simulink model "AUV_6DoF"  (R2020b)
settings: Solver=VariableStepAuto  StartTime=0.0  StopTime=60  RelTol=1e-3
libraries: pid_lib x4, simulink x1
settings Model: Creator=shanerutherford  LastModifiedBy=shanerutherford

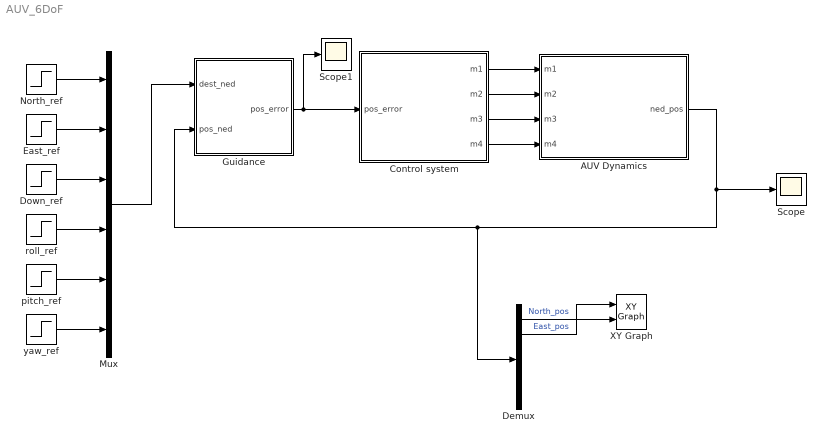
== system AUV_6DoF ==
  AUV Dynamics : Subsystem
  Control system : Subsystem
  Demux : Demux  Outputs=6
  Down_ref : Step  Time=0  After=0  SampleTime=0
  East_ref : Step  Time=0  After=-1  SampleTime=0
  Guidance : MATLAB Function  TreatAsAtomicUnit=on
  Mux : Mux  Inputs=6
  North_ref : Step  Time=0  After=-1  SampleTime=0
  Scope : Scope
  Scope1 : Scope
  XY Graph : simulink/Sinks/XY Graph  xmin=-10  xmax=10  ymin=-10  ymax=10  st=-1
  pitch_ref : Step  Time=0  After=0  SampleTime=0
  roll_ref : Step  Time=0  After=0  SampleTime=0
  yaw_ref : Step  Time=0  After=0  SampleTime=0
  wires:
  Control system/1(m1) -> AUV Dynamics/1(m1)
  Control system/2(m2) -> AUV Dynamics/2(m2)
  Control system/3(m3) -> AUV Dynamics/3(m3)
  Control system/4(m4) -> AUV Dynamics/4(m4)
  Guidance/1(pos_error) -> Scope1/1, Control system/1(pos_error)
  Mux/1 -> Guidance/1(dest_ned)
  North_ref/1 -> Mux/1
  Down_ref/1 -> Mux/3
  roll_ref/1 -> Mux/4
  yaw_ref/1 -> Mux/6
  East_ref/1 -> Mux/2
  pitch_ref/1 -> Mux/5
  AUV Dynamics/1(ned_pos) -> Scope/1, Demux/1, Guidance/2(pos_ned)
  Demux/1 -> XY Graph/2  "North_pos"
  Demux/2 -> XY Graph/1  "East_pos"

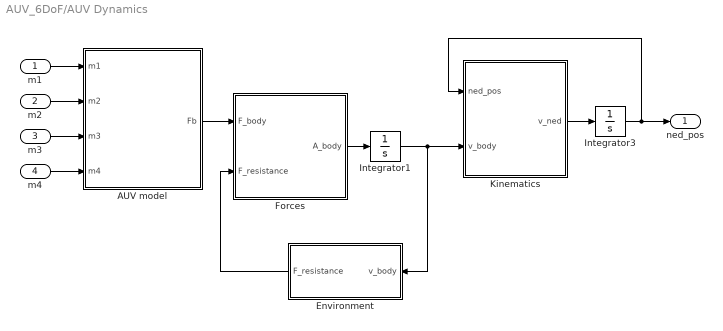
== system AUV_6DoF/AUV Dynamics ==
  m1 : Inport
  m2 : Inport  Port=2
  m3 : Inport  Port=3
  m4 : Inport  Port=4
  AUV model : MATLAB Function  TreatAsAtomicUnit=on
  Environment : MATLAB Function  TreatAsAtomicUnit=on
  Forces : MATLAB Function  TreatAsAtomicUnit=on
  Integrator1 : Integrator
  Integrator3 : Integrator
  Kinematics : MATLAB Function  TreatAsAtomicUnit=on
  ned_pos : Outport  PortDimensions=6
  wires:
  m1/1 -> AUV model/1(m1)
  m2/1 -> AUV model/2(m2)
  m3/1 -> AUV model/3(m3)
  m4/1 -> AUV model/4(m4)
  Integrator3/1 -> ned_pos/1, Kinematics/1(ned_pos)
  Kinematics/1(v_ned) -> Integrator3/1
  AUV model/1(Fb) -> Forces/1(F_body)
  Environment/1(F_resistance) -> Forces/2(F_resistance)
  Forces/1(A_body) -> Integrator1/1
  Integrator1/1 -> Kinematics/2(v_body), Environment/1(v_body)

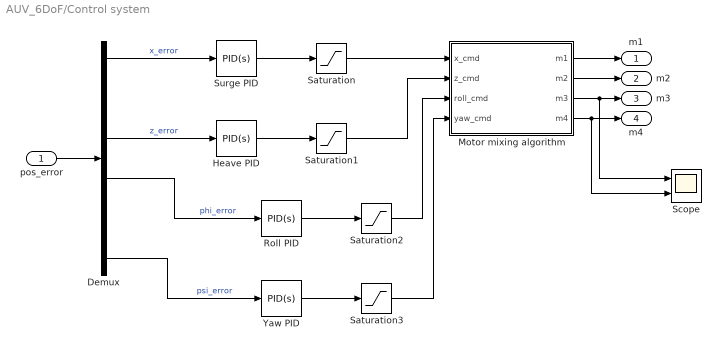
== system AUV_6DoF/Control system ==
  pos_error : Inport
  Demux : Demux  Outputs=6
  Heave PID : pid_lib/PID Controller  Controller=PID  Form=Parallel  TimeDomain=Continuous-time  UseExternalTs=off  SampleTime=-1  IntegratorMethod=Forward Euler  FilterMethod=Forward Euler  ControllerParametersSource=internal  P=1  I=0  D=5  UseFilter=on  N=100  TunerSelectOption=Transfer Function Based (PID Tuner App)  InitialConditionSource=internal  InitialConditionForIntegrator=0  InitialConditionForFilter=0  DifferentiatorICPrevScaledInput=0  ExternalReset=none  TrackingMode=off  Kt=1  LimitOutput=off  SatLimitsSource=internal  UpperSaturationLimit=inf  LowerSaturationLimit=-inf  LinearizeAsGain=on  AntiWindupMode=none  Kb=1  POutMin=[]  POutMax=[]  IOutMin=[]  IOutMax=[]  DOutMin=[]  DOutMax=[]  NOutMin=[]  NOutMax=[]  SumOutMin=[]  SumOutMax=[]  SaturationOutMin=[]  SaturationOutMax=[]  PParamMin=[]  PParamMax=[]  IParamMin=[]  IParamMax=[]  DParamMin=[]  DParamMax=[]  NParamMin=[]  NParamMax=[]  KbParamMin=[]  KbParamMax=[]  KtParamMin=[]  KtParamMax=[]  KbOutMin=[]  KbOutMax=[]  KtOutMin=[]  KtOutMax=[]  IntegratorOutMin=[]  IntegratorOutMax=[]  FilterOutMin=[]  FilterOutMax=[]  SumI1OutMin=[]  SumI1OutMax=[]  SumI2OutMin=[]  SumI2OutMax=[]  SumI3OutMin=[]  SumI3OutMax=[]  SumI4OutMin=[]  SumI4OutMax=[]  SumDOutMin=[]  SumDOutMax=[]  DifferentiatorOutMin=[]  DifferentiatorOutMax=[]  FilterDiffOutCoefMin=[]  FilterDiffOutCoefMax=[]  ReciprocalOutMin=[]  ReciprocalOutMax=[]  SumDenOutMin=[]  SumDenOutMax=[]  SumNumOutMin=[]  SumNumOutMax=[]  DivideOutMin=[]  DivideOutMax=[]  UdiffTsProdOutMin=[]  UdiffTsProdOutMax=[]  NTsProdOutMin=[]  NTsProdOutMax=[]  UintegralTsProdOutMin=[]  UintegralTsProdOutMax=[]  UngainTsProdOutMin=[]  UngainTsProdOutMax=[]  IntegratorContinuousStateAttributes=''  IntegratorStateMustResolveToSignalObject=off  IntegratorRTWStateStorageClass=Auto  FilterContinuousStateAttributes=''  FilterStateMustResolveToSignalObject=off  FilterRTWStateStorageClass=Auto  ParallelPVariant=InternalParameters  IdealPVariant=Disabled  IVariant=InternalParameters  DVariant=InternalParameters  IntegratorVariant=Continuous  SatVariant=Disabled  AWVariant=Passthrough  PCopyVariant=Disabled  TRVariant=Disabled  FdbkBlocksVariant=Forward  IdealPFdbkVariant=Disabled  SatFdbkVariant=Disabled  DerivativeFilterVariant=ContFilter  NVariant=InternalParameters  NCopyVariant=Disabled  FilterICVariant=InternalICsFilter  IntegratorICVariant=InternalICs  ExternalResetVariant=Disabled  TRSumVariant=Passthrough  SumFdbkVariant=Disabled  SumVariant=Sum_PID  TsampFilterVariant=InternalTs  TsampNgainVariant=Passthrough  TsampIntegralVariant=Passthrough  ExternalSaturationOutDataTypeStr=Inherit: Same as second input
  Motor mixing algorithm : MATLAB Function  TreatAsAtomicUnit=on
  Roll PID : pid_lib/PID Controller  Controller=PID  Form=Parallel  TimeDomain=Continuous-time  UseExternalTs=off  SampleTime=-1  IntegratorMethod=Forward Euler  FilterMethod=Forward Euler  ControllerParametersSource=internal  P=1  I=0  D=5  UseFilter=on  N=100  TunerSelectOption=Transfer Function Based (PID Tuner App)  InitialConditionSource=internal  InitialConditionForIntegrator=0  InitialConditionForFilter=0  DifferentiatorICPrevScaledInput=0  ExternalReset=none  TrackingMode=off  Kt=1  LimitOutput=off  SatLimitsSource=internal  UpperSaturationLimit=inf  LowerSaturationLimit=-inf  LinearizeAsGain=on  AntiWindupMode=none  Kb=1  POutMin=[]  POutMax=[]  IOutMin=[]  IOutMax=[]  DOutMin=[]  DOutMax=[]  NOutMin=[]  NOutMax=[]  SumOutMin=[]  SumOutMax=[]  SaturationOutMin=[]  SaturationOutMax=[]  PParamMin=[]  PParamMax=[]  IParamMin=[]  IParamMax=[]  DParamMin=[]  DParamMax=[]  NParamMin=[]  NParamMax=[]  KbParamMin=[]  KbParamMax=[]  KtParamMin=[]  KtParamMax=[]  KbOutMin=[]  KbOutMax=[]  KtOutMin=[]  KtOutMax=[]  IntegratorOutMin=[]  IntegratorOutMax=[]  FilterOutMin=[]  FilterOutMax=[]  SumI1OutMin=[]  SumI1OutMax=[]  SumI2OutMin=[]  SumI2OutMax=[]  SumI3OutMin=[]  SumI3OutMax=[]  SumI4OutMin=[]  SumI4OutMax=[]  SumDOutMin=[]  SumDOutMax=[]  DifferentiatorOutMin=[]  DifferentiatorOutMax=[]  FilterDiffOutCoefMin=[]  FilterDiffOutCoefMax=[]  ReciprocalOutMin=[]  ReciprocalOutMax=[]  SumDenOutMin=[]  SumDenOutMax=[]  SumNumOutMin=[]  SumNumOutMax=[]  DivideOutMin=[]  DivideOutMax=[]  UdiffTsProdOutMin=[]  UdiffTsProdOutMax=[]  NTsProdOutMin=[]  NTsProdOutMax=[]  UintegralTsProdOutMin=[]  UintegralTsProdOutMax=[]  UngainTsProdOutMin=[]  UngainTsProdOutMax=[]  IntegratorContinuousStateAttributes=''  IntegratorStateMustResolveToSignalObject=off  IntegratorRTWStateStorageClass=Auto  FilterContinuousStateAttributes=''  FilterStateMustResolveToSignalObject=off  FilterRTWStateStorageClass=Auto  ParallelPVariant=InternalParameters  IdealPVariant=Disabled  IVariant=InternalParameters  DVariant=InternalParameters  IntegratorVariant=Continuous  SatVariant=Disabled  AWVariant=Passthrough  PCopyVariant=Disabled  TRVariant=Disabled  FdbkBlocksVariant=Forward  IdealPFdbkVariant=Disabled  SatFdbkVariant=Disabled  DerivativeFilterVariant=ContFilter  NVariant=InternalParameters  NCopyVariant=Disabled  FilterICVariant=InternalICsFilter  IntegratorICVariant=InternalICs  ExternalResetVariant=Disabled  TRSumVariant=Passthrough  SumFdbkVariant=Disabled  SumVariant=Sum_PID  TsampFilterVariant=InternalTs  TsampNgainVariant=Passthrough  TsampIntegralVariant=Passthrough  ExternalSaturationOutDataTypeStr=Inherit: Same as second input
  Saturation{,1..3} (4 alike) : Saturate  UpperLimit=0.3  LowerLimit=-0.3
  Scope : Scope  NumInputPorts=2
  Surge PID : pid_lib/PID Controller  Controller=PID  Form=Parallel  TimeDomain=Continuous-time  UseExternalTs=off  SampleTime=-1  IntegratorMethod=Forward Euler  FilterMethod=Forward Euler  ControllerParametersSource=internal  P=1  I=0  D=5  UseFilter=on  N=100  TunerSelectOption=Transfer Function Based (PID Tuner App)  InitialConditionSource=internal  InitialConditionForIntegrator=0  InitialConditionForFilter=0  DifferentiatorICPrevScaledInput=0  ExternalReset=none  TrackingMode=off  Kt=1  LimitOutput=off  SatLimitsSource=internal  UpperSaturationLimit=inf  LowerSaturationLimit=-inf  LinearizeAsGain=on  AntiWindupMode=none  Kb=1  POutMin=[]  POutMax=[]  IOutMin=[]  IOutMax=[]  DOutMin=[]  DOutMax=[]  NOutMin=[]  NOutMax=[]  SumOutMin=[]  SumOutMax=[]  SaturationOutMin=[]  SaturationOutMax=[]  PParamMin=[]  PParamMax=[]  IParamMin=[]  IParamMax=[]  DParamMin=[]  DParamMax=[]  NParamMin=[]  NParamMax=[]  KbParamMin=[]  KbParamMax=[]  KtParamMin=[]  KtParamMax=[]  KbOutMin=[]  KbOutMax=[]  KtOutMin=[]  KtOutMax=[]  IntegratorOutMin=[]  IntegratorOutMax=[]  FilterOutMin=[]  FilterOutMax=[]  SumI1OutMin=[]  SumI1OutMax=[]  SumI2OutMin=[]  SumI2OutMax=[]  SumI3OutMin=[]  SumI3OutMax=[]  SumI4OutMin=[]  SumI4OutMax=[]  SumDOutMin=[]  SumDOutMax=[]  DifferentiatorOutMin=[]  DifferentiatorOutMax=[]  FilterDiffOutCoefMin=[]  FilterDiffOutCoefMax=[]  ReciprocalOutMin=[]  ReciprocalOutMax=[]  SumDenOutMin=[]  SumDenOutMax=[]  SumNumOutMin=[]  SumNumOutMax=[]  DivideOutMin=[]  DivideOutMax=[]  UdiffTsProdOutMin=[]  UdiffTsProdOutMax=[]  NTsProdOutMin=[]  NTsProdOutMax=[]  UintegralTsProdOutMin=[]  UintegralTsProdOutMax=[]  UngainTsProdOutMin=[]  UngainTsProdOutMax=[]  IntegratorContinuousStateAttributes=''  IntegratorStateMustResolveToSignalObject=off  IntegratorRTWStateStorageClass=Auto  FilterContinuousStateAttributes=''  FilterStateMustResolveToSignalObject=off  FilterRTWStateStorageClass=Auto  ParallelPVariant=InternalParameters  IdealPVariant=Disabled  IVariant=InternalParameters  DVariant=InternalParameters  IntegratorVariant=Continuous  SatVariant=Disabled  AWVariant=Passthrough  PCopyVariant=Disabled  TRVariant=Disabled  FdbkBlocksVariant=Forward  IdealPFdbkVariant=Disabled  SatFdbkVariant=Disabled  DerivativeFilterVariant=ContFilter  NVariant=InternalParameters  NCopyVariant=Disabled  FilterICVariant=InternalICsFilter  IntegratorICVariant=InternalICs  ExternalResetVariant=Disabled  TRSumVariant=Passthrough  SumFdbkVariant=Disabled  SumVariant=Sum_PID  TsampFilterVariant=InternalTs  TsampNgainVariant=Passthrough  TsampIntegralVariant=Passthrough  ExternalSaturationOutDataTypeStr=Inherit: Same as second input
  Yaw PID : pid_lib/PID Controller  Controller=PID  Form=Parallel  TimeDomain=Continuous-time  UseExternalTs=off  SampleTime=-1  IntegratorMethod=Forward Euler  FilterMethod=Forward Euler  ControllerParametersSource=internal  P=1  I=0  D=5  UseFilter=on  N=100  TunerSelectOption=Transfer Function Based (PID Tuner App)  InitialConditionSource=internal  InitialConditionForIntegrator=0  InitialConditionForFilter=0  DifferentiatorICPrevScaledInput=0  ExternalReset=none  TrackingMode=off  Kt=1  LimitOutput=off  SatLimitsSource=internal  UpperSaturationLimit=inf  LowerSaturationLimit=-inf  LinearizeAsGain=on  AntiWindupMode=none  Kb=1  POutMin=[]  POutMax=[]  IOutMin=[]  IOutMax=[]  DOutMin=[]  DOutMax=[]  NOutMin=[]  NOutMax=[]  SumOutMin=[]  SumOutMax=[]  SaturationOutMin=[]  SaturationOutMax=[]  PParamMin=[]  PParamMax=[]  IParamMin=[]  IParamMax=[]  DParamMin=[]  DParamMax=[]  NParamMin=[]  NParamMax=[]  KbParamMin=[]  KbParamMax=[]  KtParamMin=[]  KtParamMax=[]  KbOutMin=[]  KbOutMax=[]  KtOutMin=[]  KtOutMax=[]  IntegratorOutMin=[]  IntegratorOutMax=[]  FilterOutMin=[]  FilterOutMax=[]  SumI1OutMin=[]  SumI1OutMax=[]  SumI2OutMin=[]  SumI2OutMax=[]  SumI3OutMin=[]  SumI3OutMax=[]  SumI4OutMin=[]  SumI4OutMax=[]  SumDOutMin=[]  SumDOutMax=[]  DifferentiatorOutMin=[]  DifferentiatorOutMax=[]  FilterDiffOutCoefMin=[]  FilterDiffOutCoefMax=[]  ReciprocalOutMin=[]  ReciprocalOutMax=[]  SumDenOutMin=[]  SumDenOutMax=[]  SumNumOutMin=[]  SumNumOutMax=[]  DivideOutMin=[]  DivideOutMax=[]  UdiffTsProdOutMin=[]  UdiffTsProdOutMax=[]  NTsProdOutMin=[]  NTsProdOutMax=[]  UintegralTsProdOutMin=[]  UintegralTsProdOutMax=[]  UngainTsProdOutMin=[]  UngainTsProdOutMax=[]  IntegratorContinuousStateAttributes=''  IntegratorStateMustResolveToSignalObject=off  IntegratorRTWStateStorageClass=Auto  FilterContinuousStateAttributes=''  FilterStateMustResolveToSignalObject=off  FilterRTWStateStorageClass=Auto  ParallelPVariant=InternalParameters  IdealPVariant=Disabled  IVariant=InternalParameters  DVariant=InternalParameters  IntegratorVariant=Continuous  SatVariant=Disabled  AWVariant=Passthrough  PCopyVariant=Disabled  TRVariant=Disabled  FdbkBlocksVariant=Forward  IdealPFdbkVariant=Disabled  SatFdbkVariant=Disabled  DerivativeFilterVariant=ContFilter  NVariant=InternalParameters  NCopyVariant=Disabled  FilterICVariant=InternalICsFilter  IntegratorICVariant=InternalICs  ExternalResetVariant=Disabled  TRSumVariant=Passthrough  SumFdbkVariant=Disabled  SumVariant=Sum_PID  TsampFilterVariant=InternalTs  TsampNgainVariant=Passthrough  TsampIntegralVariant=Passthrough  ExternalSaturationOutDataTypeStr=Inherit: Same as second input
  m1 : Outport
  m2 : Outport  Port=2
  m3 : Outport  Port=3
  m4 : Outport  Port=4
  wires:
  Yaw PID/1 -> Saturation3/1
  Demux/4 -> Roll PID/1  "phi_error"
  Saturation/1 -> Motor mixing algorithm/1(x_cmd)
  Demux/3 -> Heave PID/1  "z_error"
  Roll PID/1 -> Saturation2/1
  Saturation2/1 -> Motor mixing algorithm/3(roll_cmd)
  Demux/6 -> Yaw PID/1  "psi_error"
  Saturation3/1 -> Motor mixing algorithm/4(yaw_cmd)
  Saturation1/1 -> Motor mixing algorithm/2(z_cmd)
  Surge PID/1 -> Saturation/1
  Heave PID/1 -> Saturation1/1
  Motor mixing algorithm/1(m1) -> m1/1
  Motor mixing algorithm/2(m2) -> m2/1
  Motor mixing algorithm/3(m3) -> Scope/1, m3/1
  Motor mixing algorithm/4(m4) -> Scope/2, m4/1
  Demux/1 -> Surge PID/1  "x_error"
  pos_error/1 -> Demux/1

== matlab function AUV_6DoF/Control system/Motor mixing algorithm ==
  data: x_cmd input; m1 output; z_cmd input; m2 output; m3 output; m4 output; roll_cmd input; yaw_cmd input
function [m1, m2, m3, m4] = fcn(x_cmd, z_cmd, roll_cmd, yaw_cmd)

% m1 m2 m3 and m4 are front-right, front-left, back-right and back-left
% motors respectively

    function [min] = abs_min(v1, v2)
        if abs(v1) < abs(v2) 
            min = v1;
        else
            min = v2;
        end
    end

max_response = 50;

m1 = abs_min(-z_cmd - roll_cmd, max_response);
m2 = abs_min(-z_cmd + roll_cmd, max_response);
m3 = abs_min(x_cmd - yaw_cmd, max_response);
m4 = abs_min(x_cmd + yaw_cmd, max_response);
end

== matlab function AUV_6DoF/Guidance ==
  data: dest_ned input; pos_error output; pos_ned input
function pos_error  = fcn(dest_ned, pos_ned)
    % note that x is north, y is east and z is down

    N_error = dest_ned(1)-pos_ned(1);
    E_error = dest_ned(2)-pos_ned(2);
    D_error = dest_ned(3)-pos_ned(3);

    % TODO: Check if distance from target is acceptable
    current_heading = pos_ned(6);
    desired_heading = atan2(E_error, N_error);

    % convert to body axis
    x_error = max([0, N_error*cos(current_heading)+E_error*sin(current_heading)]);
    y_error = 0;
    z_error = D_error;

    roll_error = 0;
    pitch_error = 0;
    yaw_error = desired_heading - current_heading;

    while roll_error > pi
        roll_error = roll_error - 2*pi;
    end
    while roll_error < -pi
        roll_error = roll_error + 2*pi;
    end

    while yaw_error > pi
        yaw_error = yaw_error - 2*pi;
    end
    while yaw_error < -pi
        yaw_error = yaw_error + 2*pi;
    end

    pos_error = [x_error, y_error, z_error, roll_error, pitch_error, yaw_error];
end

== matlab function AUV_6DoF/AUV Dynamics/AUV model ==
  data: Fb output; m1 input; m2 input; m3 input; m4 input
function Fb = fcn(m1, m2, m3, m4)

% x, y and z axis relates to local front (bow), starboard and down
% directions
% phi, theta and psi represents roll, pitch and yaw respectivly

% assuming that the force produced by each motor is proportonal to the
% signal voltage
thrust_constant = 1;
roll_constant = 1;
yaw_constant = 1;

Fb = [thrust_constant*(m3+m4); 
      0;                           % AUV cannot move in y direction
      -thrust_constant*(m1+m2);    % positive z is downward 
      roll_constant*(m2-m1);       % positive rotation is clockwise
      0;                           % AUV cannot pitch 
      yaw_constant*(m4-m3);
];

== matlab function AUV_6DoF/AUV Dynamics/Kinematics ==
  data: ned_pos input; v_body input; v_ned output
function v_ned = fcn(ned_pos, v_body)

% calculate Jacobian using MSS toolbox function
    [J, ~, ~] = eulerang(ned_pos(4), ned_pos(5), ned_pos(6)); 
    v_ned = J * v_body;
end

== matlab function AUV_6DoF/AUV Dynamics/Forces ==
  data: A_body output size=6; F_body input; F_resistance input
function A_body = fcn(F_body, F_resistance)

mass = 10;
A_body = (F_body - F_resistance)./mass;

== matlab function AUV_6DoF/AUV Dynamics/Environment ==
  data: F_resistance output; v_body input
function F_resistance = fcn(v_body)

F_resistance = v_body.^2;
